simulink model "ArduinoSimulink_Interface"  (R2014a)
settings: Solver=FixedStepDiscrete  SolverMode=SingleTasking  StartTime=0.0  StopTime=Inf  FixedStep=0.005  RelTol=1e-3
undefined symbols (not defined in the file): Serial_Port, Standard_Devices
libraries: rtwinlib x2
CloseFcn:
  | rtwprivate ssgencode ModelCloseRequest AIRobots_UAV_CONTROL
settings Model: SimulationMode=external  ExtModeTrigDuration=60000  BufferReuse=off  Creator=Administrator  LastModifiedBy=Wilbert
settings SolverCC: AutoInsertRateTranBlk=on  InsertRTBMode=Never (minimum delay)
settings DataIOCC: Decimation=2  MaxDataPoints=60000  SaveFormat=StructureWithTime  SignalLoggingSaveFormat=ModelDataLogs  SaveOutput=off  SignalLogging=off  DSMLogging=off  SaveTime=off
settings OptimizationCC: OptimizeBlockIOStorage=off  BufferReuse=off  GlobalBufferReuse=off  ExpressionFolding=off  ExpressionDepthLimit=2147483647  LocalBlockOutputs=off  SimCompilerOptimization=On
settings DebuggingCC: UnderspecifiedInitializationDetection=Classic  MergeDetectMultiDrivingBlocksExec=error  MultiTaskDSMMsg=warning  MultiTaskCondExecSysMsg=none  MultiTaskRateTransMsg=warning  FcnCallInpInsideContextMsg=UseLocalSettings  StateNameClashWarn=warning
settings HardwareCC: ProdBitPerInt=16  ProdBitPerPointer=8  ProdIntDivRoundTo=Zero  ProdEndianess=LittleEndian  ProdWordSize=8  ProdHWDeviceType=Atmel->AVR
settings ModelReferenceCC: UpdateModelReferenceTargets=AssumeUpToDate
settings SFSimCC: SimParseCustomCode=off
settings RTWCC: SystemTargetFile=rtwin.tlc  TemplateMakefile=rtwin.tmf  Description=Real-Time Windows Target  RTWVerbose=off  ProcessScript=rtwin_make_rtw_hook  IncludeERTFirstTime=on  RTWCompilerOptimization=On
settings CodeAppCC: MaxIdLength=95  MATLABSourceComments=on
settings RTWinTargetCC: TargetLibSuffix=_rtwin.lib  TargetPreCompLibLocation=C:\Program Files\MATLAB\R2014a\toolbox\rtw\targets\rtwin\lib\win64  RebuildAll=on

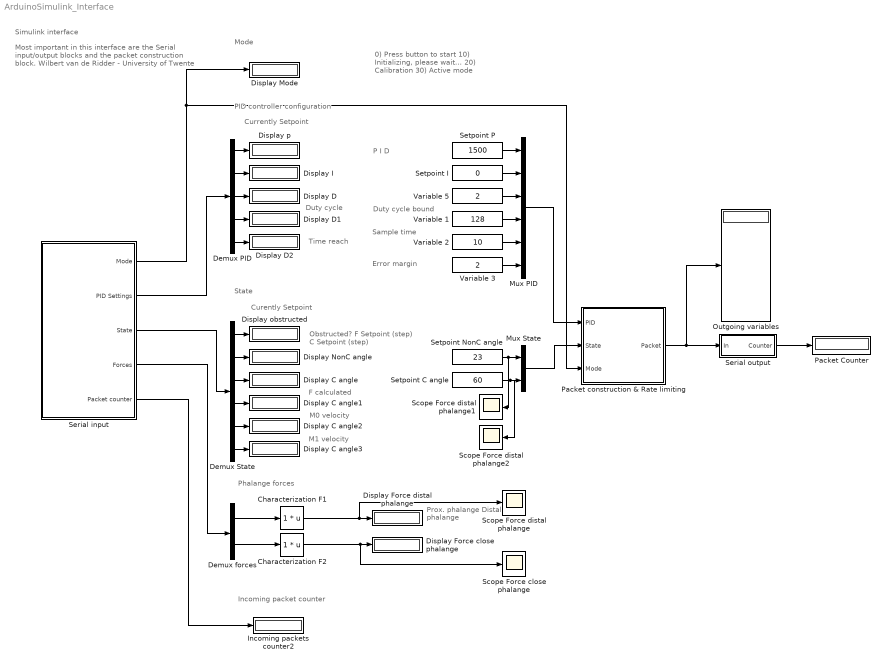
== system ArduinoSimulink_Interface ==
  note: Time reach
  note: M1 velocity
  note: M0 velocity
  note: F calculated
  note: Mode
  note: 0) Press button to start
      | 10) Initializing, please wait...
      | 20) Calibration
      | 30) Active mode
  note: Error margin
  note: Sample time
  note: Duty cycle bound
  note: Duty cycle
  note: Prox. phalange
      |
      | Distal phalange
  note: Curently Setpoint
  note: Obstructed?
      |
      | F Setpoint (step)
      |
      | C Setpoint (step)
  note: Most important in this interface are the Serial
      | input/output blocks and the packet construction
      | block.
      |
      |
      | Wilbert van de Ridder - University of Twente
  note: Currently Setpoint
  note: P
      |
      | I
      |
      | D
  note: Simulink interface
  note: Incoming packet counter
  note: PID controller configuration
  note: Phalange forces
  note: State
  Characterization F1 : Fcn  Expr=1 * u
  Characterization F2 : Fcn  Expr=1 * u
  Demux PID : Demux  Outputs=5
  Demux State : Demux  Outputs=6
  Demux forces : Demux  Outputs=2
  Display C angle{,1..3} (4 alike) : Display
  Display D : Display
  Display D1 : Display
      settings: Decimation=100
  Display D2 : Display
  Display Force close phalange : Display
  Display Force distal phalange : Display
  Display I : Display
  Display Mode : Display
  Display NonC angle : Display
  Display obstructed : Display
  Display p : Display
  Incoming packets counter2 : Display
  Mux PID : Mux  Inputs=6
  Mux State : Mux  Inputs=2
  Outgoing variables : Display
      settings: Format=bank
  Packet Counter : Display
  Packet construction & Rate limiting : Subsystem
  Scope Force close phalange : Scope
      settings: SaveName=Force2
  Scope Force distal phalange : Scope
      settings: TimeRange=60  YMin=480  YMax=620  SaveName=Force1  MaxDataPoints=50000
  Scope Force distal phalange1 : Scope
      settings: TimeRange=60  YMin=480  YMax=620  SaveName=FSetpoint
  Scope Force distal phalange2 : Scope
      settings: TimeRange=60  YMin=480  YMax=620  SaveName=CSetpoint
  Serial input : Subsystem
  Serial output : Subsystem
  Setpoint C angle : Constant  Value=60
  Setpoint I : Constant  Value=0
  Setpoint NonC angle : Constant  Value=23
  Setpoint P : Constant  Value=1500
  Variable 1 : Constant  Value=128
  Variable 2 : Constant  Value=10
  Variable 3 : Constant  Value=2
  Variable 5 : Constant  Value=2
  wires:
  Packet construction & Rate limiting/1(Packet) -> Outgoing variables/1, Serial output/1(In)
  Serial input/1(Mode) -> Display Mode/1, Packet construction & Rate limiting/3(Mode)
  Serial input/5(Packet counter) -> Incoming packets counter2/1
  Serial input/2("PID Settings ") -> Demux PID/1
  Setpoint P/1 -> Mux PID/1
  Demux PID/3 -> Display D/1
  Demux PID/2 -> Display I/1
  Setpoint I/1 -> Mux PID/2
  Variable 5/1 -> Mux PID/3
  Serial input/3(State) -> Demux State/1
  Setpoint NonC angle/1 -> Scope Force distal phalange1/1, Mux State/1
  Setpoint C angle/1 -> Scope Force distal phalange2/1, Mux State/2
  Demux State/1 -> Display obstructed/1
  Demux State/2 -> Display NonC angle/1
  Demux State/3 -> Display C angle/1
  Mux PID/1 -> Packet construction & Rate limiting/1(PID)
  Mux State/1 -> Packet construction & Rate limiting/2(State)
  Serial output/1(Counter) -> Packet Counter/1
  Serial input/4(Forces) -> Demux forces/1
  Demux forces/1 -> Characterization F1/1
  Demux forces/2 -> Characterization F2/1
  Demux PID/1 -> Display p/1
  Characterization F1/1 -> Scope Force distal phalange/1, Display Force distal phalange/1
  Characterization F2/1 -> Display Force close phalange/1, Scope Force close phalange/1
  Demux PID/4 -> Display D1/1
  Variable 2/1 -> Mux PID/5
  Variable 3/1 -> Mux PID/6
  Demux State/4 -> Display C angle1/1
  Demux State/5 -> Display C angle2/1
  Demux State/6 -> Display C angle3/1
  Variable 1/1 -> Mux PID/4
  Demux PID/5 -> Display D2/1

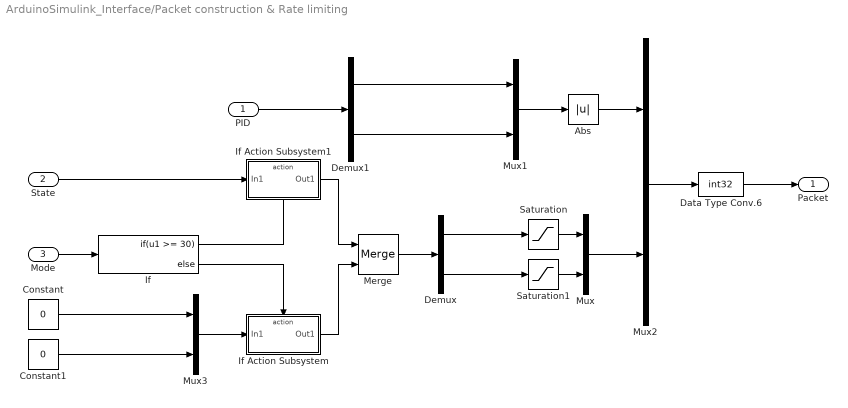
== system ArduinoSimulink_Interface/Packet construction & Rate limiting ==
  PID : Inport
  State : Inport  Port=2
  Mode : Inport  Port=3
  Abs : Abs
  Constant : Constant  Value=0
  Constant1 : Constant  Value=0
  Data Type Conv.6 : DataTypeConversion  OutDataTypeStr=int32  ConvertRealWorld=Stored Integer (SI)  RndMeth=Round
  Demux : Demux  Outputs=2
  Demux1 : Demux  Outputs=2
  If : If  IfExpression=u1 >= 30
  If Action Subsystem : Subsystem  TreatAsAtomicUnit=on
  If Action Subsystem1 : Subsystem  TreatAsAtomicUnit=on
  Merge : Merge
  Mux{,1..3} (4 alike) : Mux  Inputs=2
  Saturation : Saturate  UpperLimit=100  LowerLimit=0
  Saturation1 : Saturate  UpperLimit=100  LowerLimit=0
  Packet : Outport
  wires:
  Data Type Conv.6/1 -> Packet/1
  Mux2/1 -> Data Type Conv.6/1
  Saturation/1 -> Mux/1
  Saturation1/1 -> Mux/2
  Demux/2 -> Saturation1/1
  Demux/1 -> Saturation/1
  Mux/1 -> Mux2/2
  Merge/1 -> Demux/1
  Demux1/1 -> Mux1/1
  Demux1/2 -> Mux1/2
  Mux1/1 -> Abs/1
  PID/1 -> Demux1/1
  If/2 -> If Action Subsystem/Action
  If/1 -> If Action Subsystem1/Action
  Mode/1 -> If/1
  Constant/1 -> Mux3/1
  Constant1/1 -> Mux3/2
  State/1 -> If Action Subsystem1/1(In1)
  Mux3/1 -> If Action Subsystem/1(In1)
  If Action Subsystem1/1(Out1) -> Merge/1
  If Action Subsystem/1(Out1) -> Merge/2
  Abs/1 -> Mux2/1

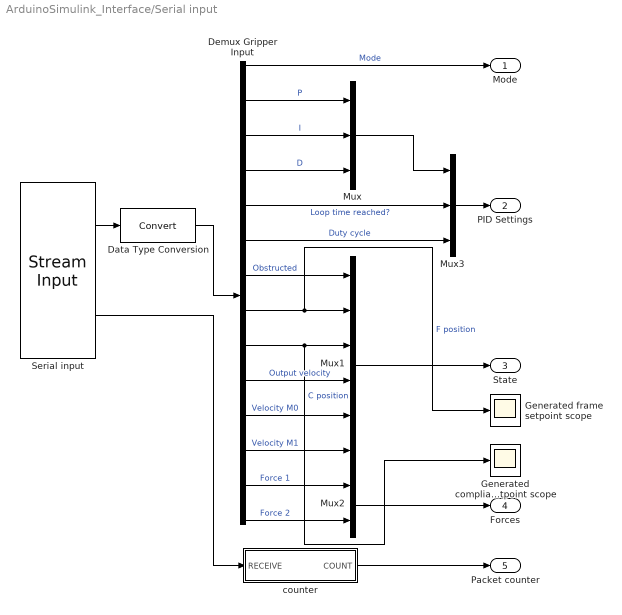
== system ArduinoSimulink_Interface/Serial input ==
  Data Type Conversion : DataTypeConversion
  Demux Gripper Input : Demux  Outputs=14
  Generated compliance setpoint scope : Scope
      settings: SaveName=CGenSetpoint1
  Generated frame setpoint scope : Scope
      settings: SaveName=FGenSetpoint
  Mux : Mux  Inputs=3
  Mux1 : Mux  Inputs=6
  Mux2 : Mux  Inputs=2
  Mux3 : Mux  Inputs=3
  Serial input : rtwinlib/Stream Input  SampleTime=0.01  MaxMissedTicks=10  ShowMissedTicks=off  YieldWhenWaiting=on  DrvName=Standard_Devices/Serial_Port  DrvAddress=3  DrvOptions=[115200 8 0 0 0 0 0 0]  DataTypes={'14*int32'}  FormatString='S %d %d %d %d %d %d %d %d %d %d %d %d %d %d E'  Terminator='\n'  ShowReady=on  ShowError=off
      settings: AttributesFormatString=Standard Devices\nSerial Port [3h]
  counter : Subsystem
  Mode : Outport
  "PID Settings " : Outport  Port=2
  State : Outport  Port=3
  Forces : Outport  Port=4
  Packet counter : Outport  Port=5
  wires:
  Serial input/1 -> Data Type Conversion/1
  Demux Gripper Input/1 -> Mode/1  "Mode"
  Demux Gripper Input/2 -> Mux/1  "P"
  Demux Gripper Input/3 -> Mux/2  "I"
  Demux Gripper Input/4 -> Mux/3  "D"
  Mux1/1 -> State/1
  Mux2/1 -> Forces/1
  counter/1(COUNT) -> Packet counter/1
  Serial input/2 -> counter/1(RECEIVE)
  Mux3/1 -> "PID Settings "/1
  Demux Gripper Input/5 -> Mux3/2  "Loop time reached?"
  Data Type Conversion/1 -> Demux Gripper Input/1
  Mux/1 -> Mux3/1
  Demux Gripper Input/6 -> Mux3/3  "Duty cycle"
  Demux Gripper Input/7 -> Mux1/1  "Obstructed"
  Demux Gripper Input/8 -> Generated frame setpoint scope/1, Mux1/2  "F position"
  Demux Gripper Input/9 -> Generated compliance setpoint scope/1, Mux1/3  "C position"
  Demux Gripper Input/10 -> Mux1/4  "Output velocity"
  Demux Gripper Input/11 -> Mux1/5  "Velocity M0"
  Demux Gripper Input/12 -> Mux1/6  "Velocity M1"
  Demux Gripper Input/13 -> Mux2/1  "Force 1"
  Demux Gripper Input/14 -> Mux2/2  "Force 2"

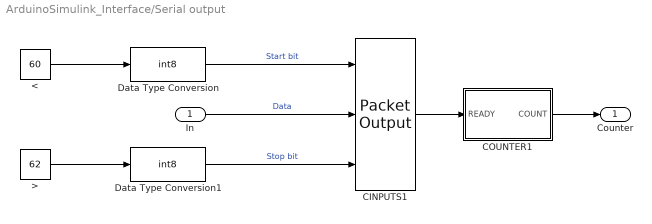
== system ArduinoSimulink_Interface/Serial output ==
  In : Inport
  < : Constant  Value=60
  > : Constant  Value=62
  CINPUTS1 : rtwinlib/Packet Output  SampleTime=0.1  MaxMissedTicks=10  ShowMissedTicks=off  YieldWhenWaiting=on  DrvName=Standard_Devices/Serial_Port  DrvAddress=3  DrvOptions=[115200 8 0 0 0 0 0 0]  PacketSize=34  DataTypes={'1*int8','8*int32', '1*int8'}  ShowReady=on  ShowError=off  PacketID=1  ByteOrder=2  InitialValue=[]  FinalValue=[]
      settings: AttributesFormatString=Standard Devices\nSerial Port [3h]
  COUNTER1 : Subsystem
  Data Type Conversion : DataTypeConversion  OutDataTypeStr=int8
  Data Type Conversion1 : DataTypeConversion  OutDataTypeStr=int8
  Counter : Outport
  wires:
  COUNTER1/1(COUNT) -> Counter/1
  CINPUTS1/1 -> COUNTER1/1(READY)
  Data Type Conversion/1 -> CINPUTS1/1  "Start bit"
  In/1 -> CINPUTS1/2  "Data"
  </1 -> Data Type Conversion/1
  Data Type Conversion1/1 -> CINPUTS1/3  "Stop bit"
  >/1 -> Data Type Conversion1/1

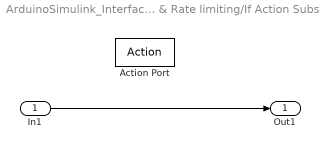
== system ArduinoSimulink_Interface/Packet construction & Rate limiting/If Action Subsystem ==
  In1 : Inport
  Action Port : ActionPort  ActionType=else
  Out1 : Outport
  wires:
  In1/1 -> Out1/1

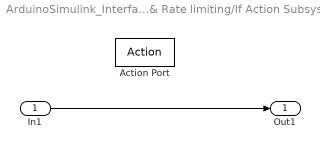
== system ArduinoSimulink_Interface/Packet construction & Rate limiting/If Action Subsystem1 ==
  In1 : Inport
  Action Port : ActionPort  ActionType=then
  Out1 : Outport
  wires:
  In1/1 -> Out1/1

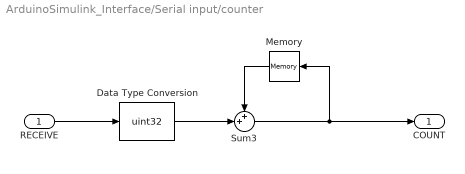
== system ArduinoSimulink_Interface/Serial input/counter ==
  RECEIVE : Inport
  Data Type Conversion : DataTypeConversion  OutDataTypeStr=uint32  LockScale=on
  Memory : Memory  InheritSampleTime=on
  Sum3 : Sum  Inputs=++|
  COUNT : Outport
  wires:
  RECEIVE/1 -> Data Type Conversion/1
  Sum3/1 -> Memory/1, COUNT/1
  Data Type Conversion/1 -> Sum3/2
  Memory/1 -> Sum3/1

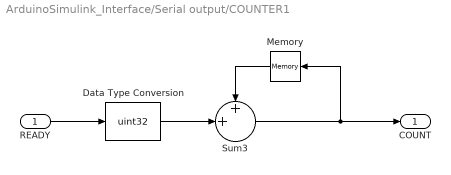
== system ArduinoSimulink_Interface/Serial output/COUNTER1 ==
  READY : Inport
  Data Type Conversion : DataTypeConversion  OutDataTypeStr=uint32  LockScale=on
  Memory : Memory  InheritSampleTime=on
  Sum3 : Sum  Inputs=++|
  COUNT : Outport
  wires:
  Sum3/1 -> Memory/1, COUNT/1
  READY/1 -> Data Type Conversion/1
  Data Type Conversion/1 -> Sum3/2
  Memory/1 -> Sum3/1
